simulink model "sim_v2"  (R2016b)
settings: Solver=FixedStepAuto  StartTime=0.0  StopTime=50  FixedStep=Ts  RelTol=1e-3
values from neighbouring files (symbols this model uses):
  initial_condition = [9 0 0 0 0 0 0 0]    [exp4_p3_2.m]    (also in exp4_p3_3.m = [pi/20 0 0 0 0 0 0 0]; exp4_p3_4.m = [pi/20 0 0 0 0 0 0 0]; exp4_p3_5.m = [pi/20 0 0 0 0 0 0 0]; exp4_p3_6.m = [pi/20 0 0 0 0 0 0 0])
  k_initial_condition = [pi/20 0 0 0 0 0 0 0]    [exp4_p3_3.m]    (also in exp4_p3_4.m; exp4_p3_5.m; exp4_p3_6.m)
  Ts = 0.0001    [exp4_p3_3.m]    (also in exp4_p3_4.m; exp4_p3_5.m; exp4_p3_6.m)
  V = [[8.6 0]; [0 3.0]]*10^-4    [exp4_p3_3.m]    (also in exp4_p3_4.m = [[8.6 0]; [0 3.0]]*10^-6; exp4_p3_5.m = [[8.6 0]; [0 3.0]]*10^-6; exp4_p3_6.m = [[8.6 0]; [0 3.0]]*10^-6)
  W = [[1.3 0]; [0 1.7]]*10^-6    [exp4_p3_3.m]    (also in exp4_p3_4.m = [[1.3 0]; [0 1.7]]*10^-3; exp4_p3_5.m = [[1.3 0]; [0 1.7]]*10^-3; exp4_p3_6.m = [[1.3 0]; [0 1.7]]*10^-3)
  y0 = [x0(1) x0(3)]    [exp4_p3_3.m]    (also in exp4_p3_4.m; exp4_p3_5.m; exp4_p3_6.m)
undefined symbols (not defined in the file or in its folder): A_0, B_0, C_0, D_0, K, L, u0, x0
libraries: simulink x2
settings Model: Creator=mariv  LastModifiedBy=mariv

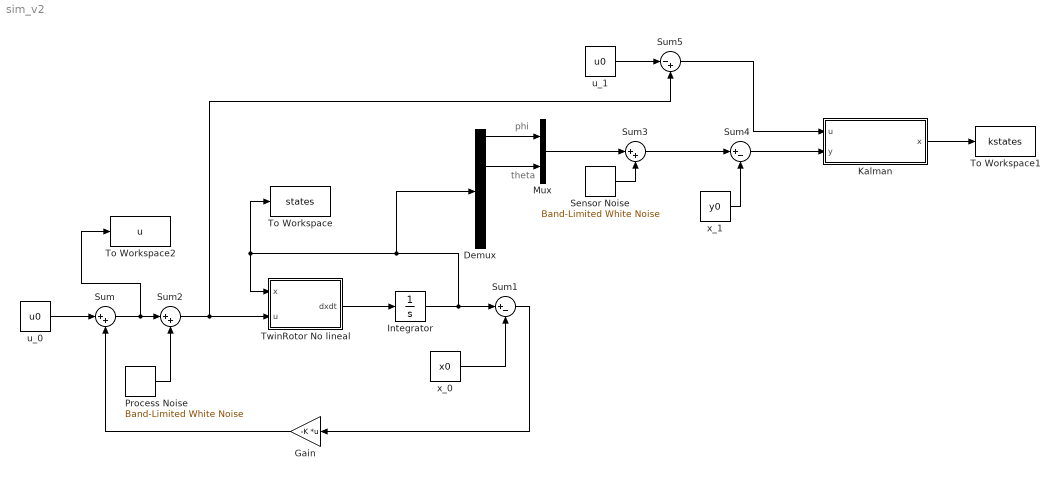
== system sim_v2 ==
  note: phi
  note: theta
  Demux : Demux  Outputs=8
  Gain : Gain  Gain=-K  Multiplication=Matrix(K*u)
  Integrator : Integrator  InitialCondition=initial_condition
  Kalman : Subsystem
  Mux : Mux  Inputs=2
  Process Noise : simulink/Sources/Band-Limited White Noise  Cov=diag(W)  Ts=Ts  seed=[23341]
  "Sensor Noise " : simulink/Sources/Band-Limited White Noise  Cov=diag(V)  Ts=Ts  seed=[23342]
  Sum : Sum  Inputs=|++
  Sum1 : Sum  Inputs=|+-
  Sum2 : Sum  Inputs=|++
  Sum3 : Sum  Inputs=|++
  Sum4 : Sum  Inputs=|+-
  Sum5 : Sum  Inputs=|-+
  To Workspace : ToWorkspace  VariableName=states  SaveFormat=Timeseries  SampleTime=-1
  To Workspace1 : ToWorkspace  VariableName=kstates  SaveFormat=Timeseries  SampleTime=-1
  To Workspace2 : ToWorkspace  VariableName=u  SaveFormat=Timeseries  SampleTime=-1
  TwinRotor No lineal : MATLAB Function  TreatAsAtomicUnit=on
  u_0 : Constant  Value=u0
  u_1 : Constant  Value=u0
  x_0 : Constant  Value=x0
  x_1 : Constant  Value=y0
  wires:
  TwinRotor No lineal/1(dxdt) -> Integrator/1
  Integrator/1 -> Sum1/1, Demux/1, To Workspace/1, TwinRotor No lineal/1(x)
  u_0/1 -> Sum/1
  x_0/1 -> Sum1/2
  Sum1/1 -> Gain/1
  Gain/1 -> Sum/2
  Demux/1 -> Mux/1
  Demux/3 -> Mux/2
  Kalman/1(x) -> To Workspace1/1
  Process Noise/1 -> Sum2/2
  Sum/1 -> To Workspace2/1, Sum2/1
  Sum2/1 -> Sum5/2, TwinRotor No lineal/2(u)
  "Sensor Noise "/1 -> Sum3/2
  Mux/1 -> Sum3/1
  Sum3/1 -> Sum4/1
  x_1/1 -> Sum4/2
  Sum4/1 -> Kalman/2(y)
  u_1/1 -> Sum5/1
  Sum5/1 -> Kalman/1(u)

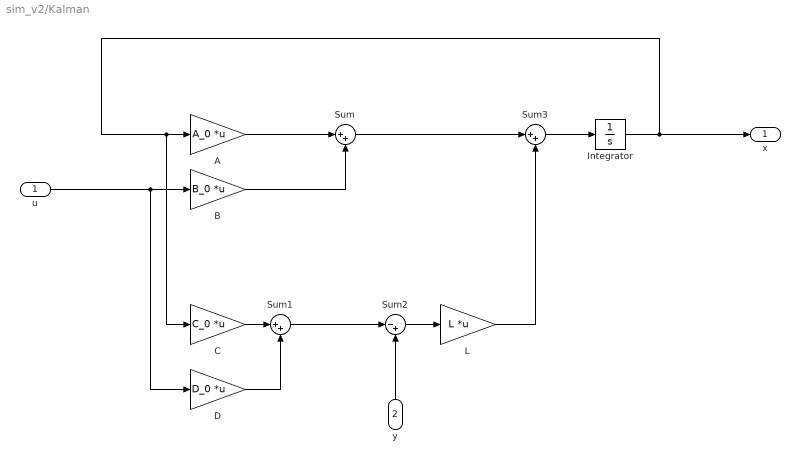
== system sim_v2/Kalman ==
  u : Inport
  y : Inport  Port=2
  A : Gain  Gain=A_0  Multiplication=Matrix(K*u)
  B : Gain  Gain=B_0  Multiplication=Matrix(K*u)
  C : Gain  Gain=C_0  Multiplication=Matrix(K*u)
  D : Gain  Gain=D_0  Multiplication=Matrix(K*u)
  Integrator : Integrator  InitialCondition=k_initial_condition
  L : Gain  Gain=L  Multiplication=Matrix(K*u)
  Sum : Sum  Inputs=|++
  Sum1 : Sum  Inputs=|++
  Sum2 : Sum  Inputs=|-+
  Sum3 : Sum  Inputs=|++
  x : Outport
  wires:
  Integrator/1 -> C/1, A/1, x/1
  u/1 -> D/1, B/1
  A/1 -> Sum/1
  B/1 -> Sum/2
  C/1 -> Sum1/1
  D/1 -> Sum1/2
  y/1 -> Sum2/2
  Sum1/1 -> Sum2/1
  Sum2/1 -> L/1
  Sum/1 -> Sum3/1
  L/1 -> Sum3/2
  Sum3/1 -> Integrator/1

== matlab function sim_v2/TwinRotor No lineal ==
  data: x input; u input; dxdt output
function dxdt = fcn(x, u)
phi = x(1);d_phi = x(2);theta = x(3);d_theta = x(4);w_p = x(5); w_t = x(6); i_p = x(7); i_t = x(8);
u_p = u(1); u_t = u(2);
dxdt = [d_phi;
(((2231553*cos(phi)^2)/4000000 + 6271303914229987/36028797018963968)*((3*d_phi)/250 - (27043227*cos(phi))/20000000 + (3022461*sin(phi))/2500000 + (1256252657407189*d_theta^2*sin(2*phi))/9007199254740992 + (2921964261275593*w_p*abs(w_p))/9223372036854775808))/((1566754414544131*cos(phi)*sin(phi))/9223372036854775808 - (1850992331451507*cos(phi)^2)/9007199254740992 + (3504602316272157*sin(phi)^2)/36893488147419103232 - 4621850957490069/72057594037927936) - (((1027*cos(phi))/25000 + (9189*sin(phi))/200000)*((6466506135038883*w_t*abs(w_t))/368934881474191032320 - (9*d_theta)/5000 + (9*d_phi^2*((9189*cos(phi))/200000 - (1027*sin(phi))/25000))/200 + (1507503188888627*d_phi*d_theta*sin(2*phi))/18014398509481984 + (7304910653188983*w_p*abs(w_p)*sin(phi))/368934881474191032320))/((1566754414544131*cos(phi)*sin(phi))/9223372036854775808 - (1850992331451507*cos(phi)^2)/9007199254740992 + (3504602316272157*sin(phi)^2)/36893488147419103232 - 4621850957490069/72057594037927936);
d_theta;
(((1027*cos(phi))/25000 + (9189*sin(phi))/200000)*((9*d_phi)/2500 - (81129681*cos(phi))/200000000 + (9067383*sin(phi))/25000000 + (1507503188888627*d_theta^2*sin(2*phi))/36028797018963968 + (438294639191339*w_p*abs(w_p))/4611686018427387904))/((1566754414544131*cos(phi)*sin(phi))/9223372036854775808 - (1850992331451507*cos(phi)^2)/9007199254740992 + (3504602316272157*sin(phi)^2)/36893488147419103232 - 4621850957490069/72057594037927936) - ((3177141253833869*w_t*abs(w_t))/73786976294838206464 - (4978621639436999*d_theta)/1125899906842624000 + (4978621639436999*d_phi^2*((9189*cos(phi))/200000 - (1027*sin(phi))/25000))/45035996273704960 + (7406705370233703*d_phi*d_theta*sin(2*phi))/36028797018963968 + (7178136850767151*w_p*abs(w_p)*sin(phi))/147573952589676412928)/((1566754414544131*cos(phi)*sin(phi))/9223372036854775808 - (1850992331451507*cos(phi)^2)/9007199254740992 + (3504602316272157*sin(phi)^2)/36893488147419103232 - 4621850957490069/72057594037927936);
(74600*i_p)/1083 - (300*w_p)/361;
(1492000*i_t)/10609 - (8000*w_t)/10609;
(25000*u_p)/21 - (75000*i_p)/7 - (1865*w_p)/21;
(25000*u_t)/21 - (75000*i_t)/7 - (1865*w_t)/21;
];
